simulink model "Clutch_lock_up_model"  (R2020b)
settings: Solver=VariableStepAuto  StartTime=0.0  StopTime=10.0  RelTol=1e-3
undefined symbols (not defined in the file or in its folder): be, bv, Ie, Iv, R, Uk, Us
settings Model: Creator=JAGRUTI SHINDE  LastModifiedBy=JAGRUTI SHINDE

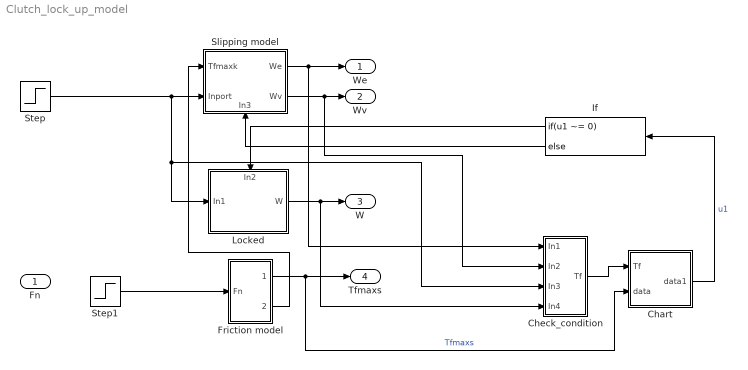
== system Clutch_lock_up_model ==
  Fn : Inport
  Chart : Stateflow chart  TreatAsAtomicUnit=on
  Check_condition : Subsystem
  Friction model : Subsystem
  If : If  IfExpression=u1 ~= 0
  Locked : Subsystem
      settings: PortSchema="{\"entries\":[{\"content\":{\"sides\":[{\"content\":{\"connectorIds\":[\"In1\"]},\"type\":\"ConnectorPlacement.EquallySpacedRectSide\",\"uuid\":\"d680e90a-3d05-4b07-99af-ba9d3634b971\"},{\"content\":{\"connectorIds\":[\"Out1\"],\"side\":\"RIGHT\"},\"type\":\"ConnectorPlacement.EquallySpacedRectSide\",\"uuid\":\"2f7bce8f-7a15-4a85-b869-386858cb7efc\"},{\"content\":{\"connectorIds\":[\"In2\"],\"side\":\"TOP\"},\"type\":\"ConnectorPlacement.EquallySpacedRectSide\",\"uuid\":\"e1e3c273-9103-4941-8a86-44507270f091\"},{\"content\":{\"connectorIds\":[],\"side\":\"HIDDEN\"},\"type\":\"ConnectorPlacement.EquallySpacedRectSide\",\"uuid\":\"ceee5c52-701a-41aa-8411-62ef9acab660\"}]},\"type\":\"ConnectorPlacement.EquallySpacedConnector\",\"uuid\":\"a783f40a-3566-47e3-bc49-041a27b862f6\"}],\"packageUris\":[\"http://schema.mathworks.com/mf0/Connector/R2020b\"],\"version\":\"1.0\"}"
  Slipping model : Subsystem
      settings: PortSchema="{\"entries\":[{\"content\":{\"sides\":[{\"content\":{\"connectorIds\":[\"In1\",\"In2\"]},\"type\":\"ConnectorPlacement.EquallySpacedRectSide\",\"uuid\":\"8019448e-cc9c-4152-aad9-a60801cc60cd\"},{\"content\":{\"connectorIds\":[\"Out1\",\"Out2\"],\"side\":\"RIGHT\"},\"type\":\"ConnectorPlacement.EquallySpacedRectSide\",\"uuid\":\"6375becc-a18f-44c7-b5b2-8427141f2704\"},{\"content\":{\"connectorIds\":[],\"side\":\"TOP\"},\"type\":\"ConnectorPlacement.EquallySpacedRectSide\",\"uuid\":\"6623764c-5dfb-4a0c-8499-8a2a6779b64e\"},{\"content\":{\"connectorIds\":[\"In3\"],\"side\":\"BOTTOM\"},\"type\":\"ConnectorPlacement.EquallySpacedRectSide\",\"uuid\":\"3840ca4e-2848-410b-a468-0a20b7caee11\"},{\"content\":{\"connectorIds\":[],\"side\":\"HIDDEN\"},\"type\":\"ConnectorPlacement.EquallySpacedRectSide\",\"uuid\":\"ee356ed0-69cc-4a6b-a3b6-8b5b6e5d18a9\"}]},\"type\":\"ConnectorPlacement.EquallySpacedConnector\",\"uuid\":\"ba8e2f7d-cda4-487f-934d-c48b11ba8937\"}],\"packageUris\":[\"http://schema.mathworks.com/mf0/Connector/R2020b\"],\"version\":\"1.0\"}"
  Step : Step  SampleTime=0
  Step1 : Step  Time=5  SampleTime=0
  We : Outport
  Wv : Outport  Port=2
  W : Outport  Port=3
  Tfmaxs : Outport  Port=4
  wires:
  Friction model/2(Tfmaxk) -> Slipping model/1(Tfmaxk)
  Slipping model/1(We) -> Check_condition/1(In1), We/1
  Slipping model/2(Wv) -> Check_condition/2(In2), Wv/1
  Step/1 -> Check_condition/3(In3), Locked/1(In1), Slipping model/2(Inport)
  Locked/1(W) -> Check_condition/4(In4), W/1
  Step1/1 -> Friction model/1(Fn)
  Friction model/1(Tfmaxs) -> Chart/2(data), Tfmaxs/1  "Tfmaxs"
  If/1 -> Locked/2(In2)
  If/2 -> Slipping model/3(In3)
  Check_condition/1(Tf) -> Chart/1(Tf)
  Chart/1(data1) -> If/1  "u1"

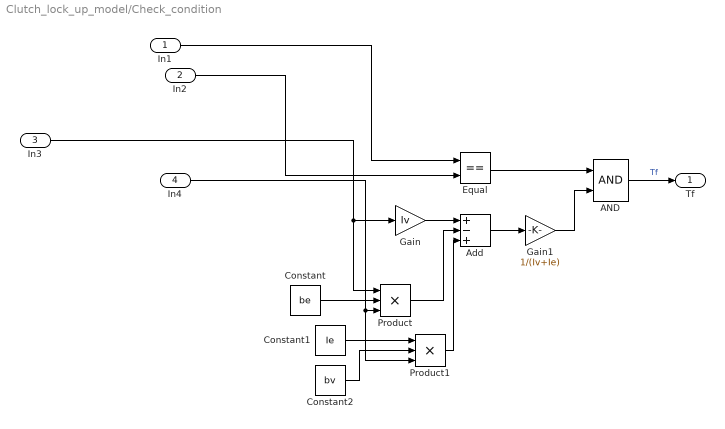
== system Clutch_lock_up_model/Check_condition ==
  In1 : Inport
  In2 : Inport  Port=2
  In3 : Inport  Port=3
  In4 : Inport  Port=4
  AND : Logic  IconShape=distinctive  AllPortsSameDT=off  OutDataTypeStr=boolean
  Add : Sum  Inputs=+-+
  Constant : Constant  Value=be
  Constant1 : Constant  Value=Ie
  Constant2 : Constant  Value=bv
  Equal : RelationalOperator  Operator===  OutDataTypeStr=boolean  RndMeth=Simplest
  Gain : Gain  Gain=Iv
  Gain1 : Gain  Gain=1/(Iv+Ie)
  Product : Product  Inputs=3
  Product1 : Product  Inputs=3
  Tf : Outport
  wires:
  In4/1 -> Product1/3, Product/3
  Equal/1 -> AND/1
  In3/1 -> Product/1, Gain/1
  Gain/1 -> Add/1
  Product/1 -> Add/2
  Constant2/1 -> Product1/2
  AND/1 -> Tf/1  "Tf"
  Constant1/1 -> Product1/1
  Constant/1 -> Product/2
  Product1/1 -> Add/3
  Gain1/1 -> AND/2
  Add/1 -> Gain1/1
  In2/1 -> Equal/2
  In1/1 -> Equal/1

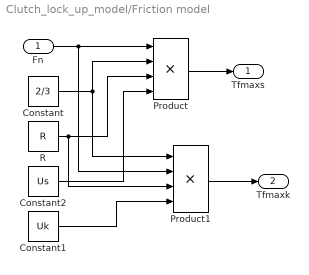
== system Clutch_lock_up_model/Friction model ==
  Fn : Inport
  Constant : Constant  Value=2/3
  Constant1 : Constant  Value=Uk
  Constant2 : Constant  Value=Us
  Product : Product  Inputs=4
  Product1 : Product  Inputs=4
  R : Constant  Value=R
  Tfmaxs : Outport
  Tfmaxk : Outport  Port=2
  wires:
  Product1/1 -> Tfmaxk/1
  Constant/1 -> Product1/1, Product/2
  R/1 -> Product1/3, Product/3
  Constant1/1 -> Product1/4
  Fn/1 -> Product1/2, Product/1
  Constant2/1 -> Product/4
  Product/1 -> Tfmaxs/1

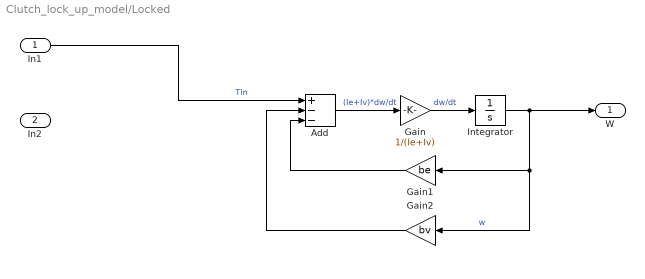
== system Clutch_lock_up_model/Locked ==
  In1 : Inport
  In2 : Inport  Port=2
  Add : Sum  Inputs=+--
  Gain : Gain  Gain=1/(Ie+Iv)
  Gain1 : Gain  Gain=be
  Gain2 : Gain  Gain=bv
  Integrator : Integrator
  W : Outport
  wires:
  Integrator/1 -> W/1, Gain2/1, Gain1/1  "w"
  Add/1 -> Gain/1  "(Ie+Iv)*dw/dt"
  Gain1/1 -> Add/3
  Gain2/1 -> Add/2
  Gain/1 -> Integrator/1  "dw/dt"
  In1/1 -> Add/1  "Tin"

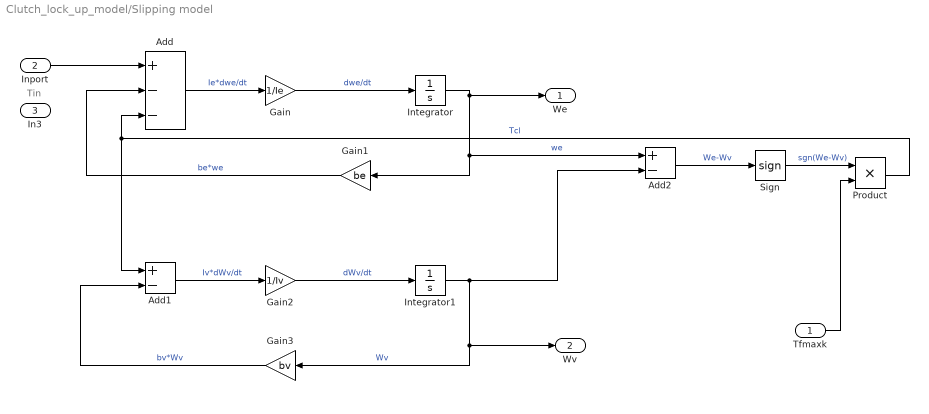
== system Clutch_lock_up_model/Slipping model ==
  note: Tin
  Tfmaxk : Inport
  Inport : Inport  Port=2
  In3 : Inport  Port=3
  Add : Sum  Inputs=+--
  Add1 : Sum  Inputs=+-
  Add2 : Sum  Inputs=+-
  Gain : Gain  Gain=1/Ie
  Gain1 : Gain  Gain=be
  Gain2 : Gain  Gain=1/Iv
  Gain3 : Gain  Gain=bv
  Integrator : Integrator
  Integrator1 : Integrator
  Product : Product
  Sign : Signum
  We : Outport
  Wv : Outport  Port=2
  wires:
  Add2/1 -> Sign/1  "We-Wv"
  Gain/1 -> Integrator/1  "dwe/dt"
  Product/1 -> Add1/1, Add/3  "Tcl"
  Integrator/1 -> We/1, Gain1/1, Add2/1  "we"
  Integrator1/1 -> Add2/2, Wv/1, Gain3/1  "Wv"
  Tfmaxk/1 -> Product/2
  Sign/1 -> Product/1  "sgn(We-Wv)"
  Add/1 -> Gain/1  "Ie*dwe/dt"
  Inport/1 -> Add/1
  Add1/1 -> Gain2/1  "Iv*dWv/dt"
  Gain2/1 -> Integrator1/1  "dWv/dt"
  Gain1/1 -> Add/2  "be*we"
  Gain3/1 -> Add1/2  "bv*Wv"

== stateflow chart Clutch_lock_up_model/Chart ==
  state Unlock
    data1=0
  state locked
    data1=1
  (default) -> Unlock
  Unlock -> locked : [Tf<=data]
  locked -> Unlock : [Tf>data]
  data: Tf input; data input; data1 output
